simulink model "phase2_soc_tasks"  (R2026a)
settings: Solver=FixedStepDiscrete  EnableMultiTasking=on
settings Model: Creator=The MathWorks, Inc.  LastModifiedBy=rayyu
settings SolverCC: PositivePriorityOrder=on
settings HardwareCC: ProdBitPerLong=64.0  ProdLargestAtomicInteger=LongLong  ProdLargestAtomicFloat=Double  ProdHWDeviceType=ARM Compatible->ARM Cortex-A (64-bit)  HardwareBoardFeatureSet=SoCBlockset
settings RTWCC: SystemTargetFile=ert.tlc  HardwareBoard=Xilinx Zynq UltraScale+ MPSoC ZCU102 Evaluation Kit  TLCOptions="-aInlineSetEventsForThisBaseRateFcn=TLC_FALSE -aSuppressMultiTaskScheduler=TLC_FALSE  -aRateBasedStepFcn=0"  GenerateReport=on  Toolchain=Linaro AArch64 Linux v6.3.1  IncludeHyperlinkInReport=on  LaunchReport=on  GenerateTraceInfo=on  GenerateTraceReport=on  GenerateTraceReportSl=on  GenerateTraceReportSf=on  GenerateTraceReportEml=on  Description=Embedded Coder
settings ERTTargetCC: ExtModeTransport=2.0  DynamicArrayContainerType=coder::array

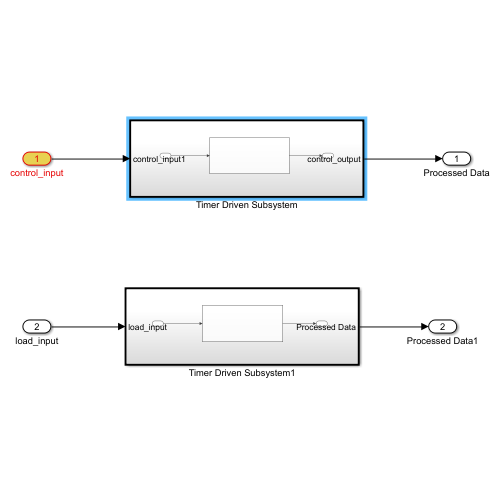
[thumbnail: Simulink's stored preview of the top-level diagram]
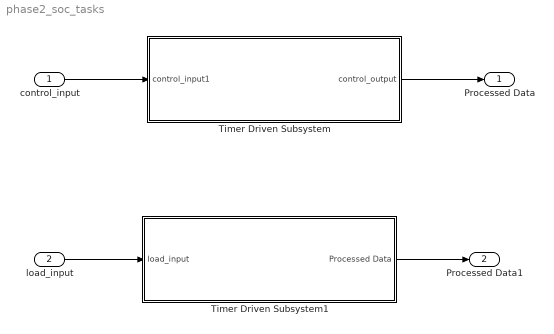
== system phase2_soc_tasks ==
  control_input : Inport
  load_input : Inport  Port=2
  Timer Driven Subsystem : Subsystem  TreatAsAtomicUnit=on
  Timer Driven Subsystem1 : Subsystem  TreatAsAtomicUnit=on
  Processed Data : Outport  VectorParamsAs1DForOutWhenUnconnected=off
  Processed Data1 : Outport  Port=2  VectorParamsAs1DForOutWhenUnconnected=off
  wires:
  Timer Driven Subsystem/1(control_output) -> Processed Data/1
  control_input/1 -> Timer Driven Subsystem/1(control_input1)
  load_input/1 -> Timer Driven Subsystem1/1(load_input)
  Timer Driven Subsystem1/1(Processed Data) -> Processed Data1/1

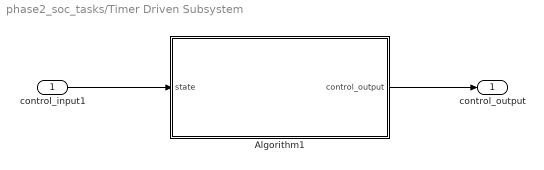
== system phase2_soc_tasks/Timer Driven Subsystem ==
  control_input1 : Inport  SampleTime=0.01
  Algorithm1 : Subsystem
  control_output : Outport  VectorParamsAs1DForOutWhenUnconnected=off
  wires:
  Algorithm1/1(control_output) -> control_output/1
  control_input1/1 -> Algorithm1/1(state)

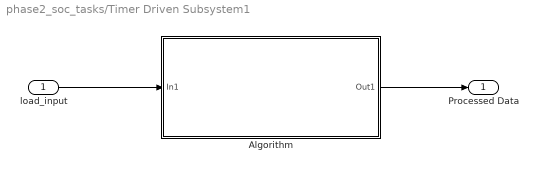
== system phase2_soc_tasks/Timer Driven Subsystem1 ==
  load_input : Inport  SampleTime=0.05
  Algorithm : Subsystem
  Processed Data : Outport  VectorParamsAs1DForOutWhenUnconnected=off
  wires:
  Algorithm/1(Out1) -> Processed Data/1
  load_input/1 -> Algorithm/1(In1)

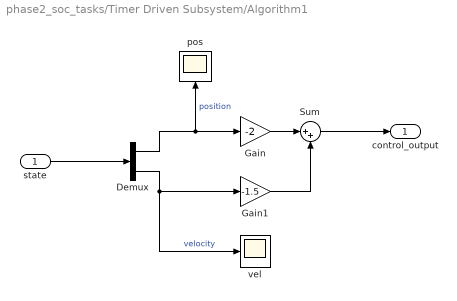
== system phase2_soc_tasks/Timer Driven Subsystem/Algorithm1 ==
  state : Inport
  Demux : Demux  Outputs=2
  Gain : Gain  Gain=-2
  Gain1 : Gain  Gain=-1.5
  Sum : Sum  Inputs=|++
  pos : Scope
      settings: ActiveDisplayYMinimum=0.97933239858184118  ActiveDisplayYMaximum=1.0022964001575732
  vel : Scope
      settings: ActiveDisplayYMinimum=-0.28436863626504516  ActiveDisplayYMaximum=0.031596515140560569
  control_output : Outport
  wires:
  Gain/1 -> Sum/1
  state/1 -> Demux/1
  Demux/1 -> Gain/1, pos/1  "position"
  Demux/2 -> Gain1/1, vel/1  "velocity"
  Gain1/1 -> Sum/2
  Sum/1 -> control_output/1

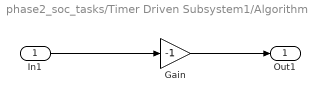
== system phase2_soc_tasks/Timer Driven Subsystem1/Algorithm ==
  In1 : Inport
  Gain : Gain  Gain=-1
  Out1 : Outport  VectorParamsAs1DForOutWhenUnconnected=off
  wires:
  In1/1 -> Gain/1
  Gain/1 -> Out1/1
